simulink library "Pitch_Functions"  (Simulink 6.5)
undefined symbols (not defined in the file or in its folder): A, ABS, B, C, D, P_PitchProfilerAccLim, P_PitchProfilerMaxGain, P_PitchProfilerPostDelay, P_PitchProfilerPreDelay, P_PitchProfilerSpdLim, P_PitchProfilerTc, P_PitchProfilerTcRatio, P_PitchSpinningPos, PITCH_CYCLE_TIME, RND, SQR
libraries: StandardLib x187, WindLib x15, Pitch_Functions x6, simulink x4
(part 3 of 3)

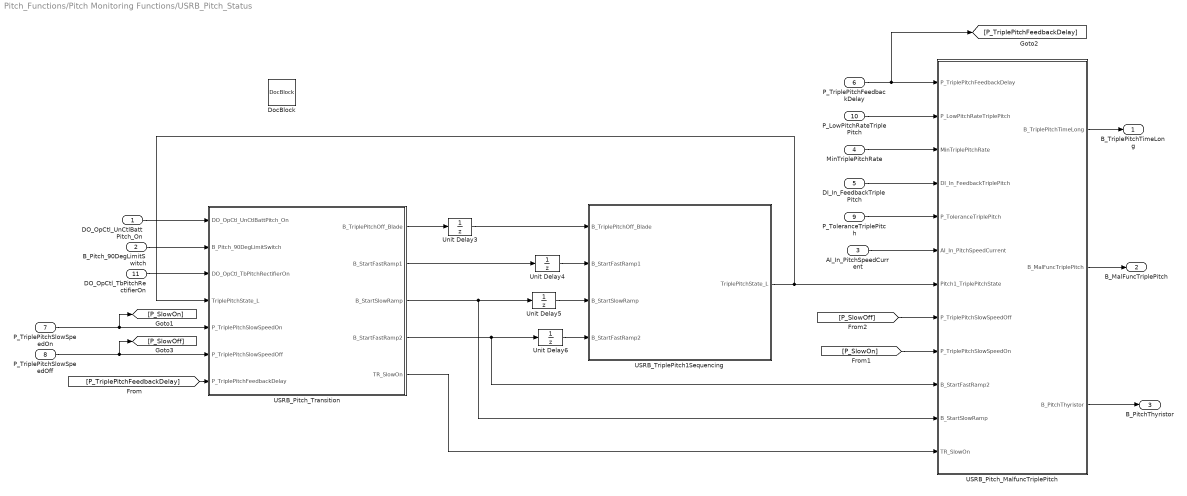
== system Pitch_Functions/Pitch Monitoring Functions/USRB_Pitch_Status ==
  DO_OpCtl_UnCtlBattPitch_On : Inport  DataType=boolean
  B_Pitch_90DegLimitSwitch : Inport  Port=2  DataType=boolean
  AI_In_PitchSpeedCurrent : Inport  Port=3  DataType=single
  MinTriplePitchRate : Inport  Port=4  DataType=single
  DI_In_FeedbackTriplePitch : Inport  Port=5  DataType=boolean
  P_TriplePitchFeedbackDelay : Inport  Port=6  DataType=uint32
  P_TriplePitchSlowSpeedOn : Inport  Port=7  DataType=uint32
  P_TriplePitchSlowSpeedOff : Inport  Port=8  DataType=uint32
  P_ToleranceTriplePitch : Inport  Port=9  DataType=single
  P_LowPitchRateTriplePitch : Inport  Port=10  DataType=single
  DO_OpCtl_TbPitchRectifierOn : Inport  Port=11  DataType=boolean
  DocBlock : simulink/Model-Wide Utilities/DocBlock  SystemSampleTime=-1  DocumentType=Text
  USRB_Pitch_MalfuncTriplePitch : Subsystem  TreatAsAtomicUnit=on
  USRB_Pitch_Transition : Subsystem  TreatAsAtomicUnit=on
  USRB_TriplePitch1Sequencing : Stateflow chart  TreatAsAtomicUnit=on
  Unit Delay{3..6} (4 alike) : UnitDelay  SampleTime=-1
  B_TriplePitchTimeLong : Outport  DataType=boolean
  B_MalFuncTriplePitch : Outport  Port=2  DataType=boolean
  B_PitchThyristor : Outport  Port=3  DataType=boolean
  wires:
  DO_OpCtl_UnCtlBattPitch_On/1 -> USRB_Pitch_Transition/1(DO_OpCtl_UnCtlBattPitch_On)
  B_Pitch_90DegLimitSwitch/1 -> USRB_Pitch_Transition/2(B_Pitch_90DegLimitSwitch)
  DO_OpCtl_TbPitchRectifierOn/1 -> USRB_Pitch_Transition/3(DO_OpCtl_TbPitchRectifierOn)
  P_TriplePitchSlowSpeedOn/1 -> USRB_Pitch_Transition/5(P_TriplePitchSlowSpeedOn), [P_SlowOn]
  P_TriplePitchSlowSpeedOff/1 -> USRB_Pitch_Transition/6(P_TriplePitchSlowSpeedOff), [P_SlowOff]
  MinTriplePitchRate/1 -> USRB_Pitch_MalfuncTriplePitch/3(MinTriplePitchRate)
  AI_In_PitchSpeedCurrent/1 -> USRB_Pitch_MalfuncTriplePitch/6(AI_In_PitchSpeedCurrent)
  P_LowPitchRateTriplePitch/1 -> USRB_Pitch_MalfuncTriplePitch/2(P_LowPitchRateTriplePitch)
  DI_In_FeedbackTriplePitch/1 -> USRB_Pitch_MalfuncTriplePitch/4(DI_In_FeedbackTriplePitch)
  P_ToleranceTriplePitch/1 -> USRB_Pitch_MalfuncTriplePitch/5(P_ToleranceTriplePitch)
  USRB_Pitch_Transition/2(B_StartFastRamp1) -> Unit Delay4/1
  USRB_Pitch_Transition/3(B_StartSlowRamp) -> USRB_Pitch_MalfuncTriplePitch/11(B_StartSlowRamp), Unit Delay5/1
  USRB_TriplePitch1Sequencing/1(TriplePitchState_L) -> USRB_Pitch_Transition/4(TriplePitchState_L), USRB_Pitch_MalfuncTriplePitch/7(Pitch1_TriplePitchState)
  USRB_Pitch_Transition/4(B_StartFastRamp2) -> USRB_Pitch_MalfuncTriplePitch/10(B_StartFastRamp2), Unit Delay6/1
  [P_TriplePitchFeedbackDelay] -> USRB_Pitch_Transition/7(P_TriplePitchFeedbackDelay)
  [P_SlowOn] -> USRB_Pitch_MalfuncTriplePitch/9(P_TriplePitchSlowSpeedOn)
  [P_SlowOff] -> USRB_Pitch_MalfuncTriplePitch/8(P_TriplePitchSlowSpeedOff)
  USRB_Pitch_MalfuncTriplePitch/1(B_TriplePitchTimeLong) -> B_TriplePitchTimeLong/1
  USRB_Pitch_MalfuncTriplePitch/2(B_MalFuncTriplePitch) -> B_MalFuncTriplePitch/1
  USRB_Pitch_MalfuncTriplePitch/3(B_PitchThyristor) -> B_PitchThyristor/1
  P_TriplePitchFeedbackDelay/1 -> USRB_Pitch_MalfuncTriplePitch/1(P_TriplePitchFeedbackDelay), [P_TriplePitchFeedbackDelay]
  USRB_Pitch_Transition/5(TR_SlowOn) -> USRB_Pitch_MalfuncTriplePitch/12(TR_SlowOn)
  Unit Delay4/1 -> USRB_TriplePitch1Sequencing/2(B_StartFastRamp1)
  Unit Delay5/1 -> USRB_TriplePitch1Sequencing/3(B_StartSlowRamp)
  Unit Delay6/1 -> USRB_TriplePitch1Sequencing/4(B_StartFastRamp2)
  USRB_Pitch_Transition/1(B_TriplePitchOff_Blade) -> Unit Delay3/1
  Unit Delay3/1 -> USRB_TriplePitch1Sequencing/1(B_TriplePitchOff_Blade)

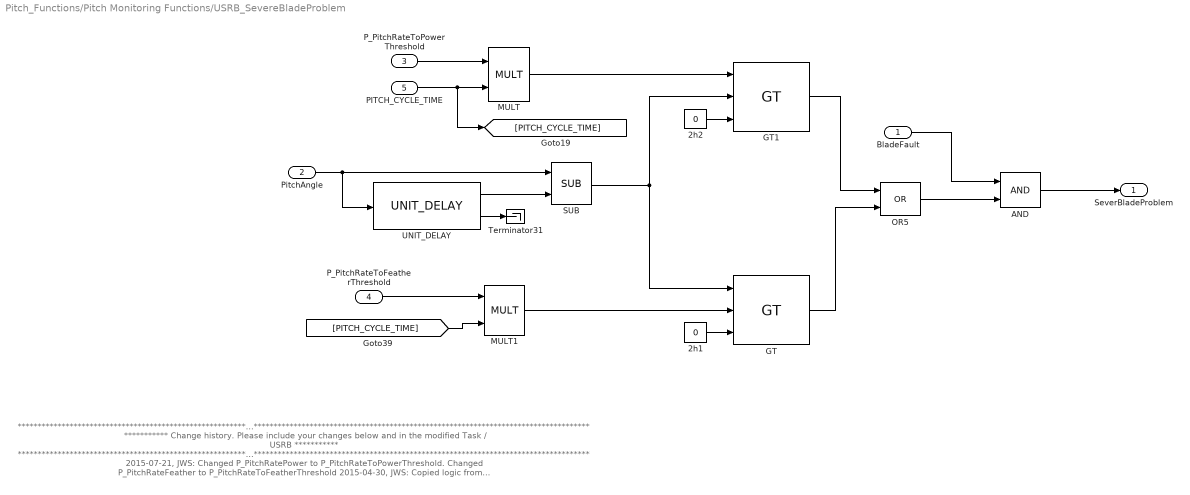
== system Pitch_Functions/Pitch Monitoring Functions/USRB_SevereBladeProblem ==
  note: ***********************************************************************************************************************************************
      | ***********         Change history. Please include your changes below and in the modified Task / USRB         ***********
      | ***********************************************************************************************************************************************
      | 2015-07-21, JWS: Changed P_PitchRatePower to P_PitchRateToPowerThreshold.
      |                             Changed P_PitchRateFeather to P_PitchRateToFeatherThreshold
      | 2015-04-30, JWS: Copied logic from Pitch_TASK_Libs.  Replaced PITCH_CYCLE_TIME constant with input.
      |                               Swapped intputs into SUB block.
  BladeFault : Inport  DataType=boolean
  PitchAngle : Inport  Port=2  DataType=single
  P_PitchRateToPowerThreshold : Inport  Port=3  DataType=single
  P_PitchRateToFeatherThreshold : Inport  Port=4  DataType=single
  PITCH_CYCLE_TIME : Inport  Port=5  DataType=single
  2h1 : Constant  Value=0  OutDataTypeMode=single  OutDataType=sfix(16)  ConRadixGroup=Use specified scaling  OutScaling=2^0  SampleTime=inf  FramePeriod=inf
  2h2 : Constant  Value=0  OutDataTypeMode=single  OutDataType=sfix(16)  ConRadixGroup=Use specified scaling  OutScaling=2^0  SampleTime=inf  FramePeriod=inf
  AND : StandardLib/Logical operations/AND  RepeatCnt=1  SampleTime=-1  ExecutionOrder=0
  GT : StandardLib/Math operations/GT  Equation=>  DataType=SINGLE  SampleTime=-1  ExecutionOrder=0
  GT1 : StandardLib/Math operations/GT  Equation=>  DataType=SINGLE  SampleTime=-1  ExecutionOrder=0
  MULT : StandardLib/Math operations/MULT  DataType=SINGLE  RepeatCnt=1  SampleTime=-1  ExecutionOrder=0
  MULT1 : StandardLib/Math operations/MULT  DataType=SINGLE  RepeatCnt=1  SampleTime=-1  ExecutionOrder=0
  OR5 : StandardLib/Logical operations/OR  RepeatCnt=1  SampleTime=-1  ExecutionOrder=0
  SUB : StandardLib/Math operations/SUB  DataType=SINGLE  SampleTime=-1  ExecutionOrder=0
  Terminator31 : Terminator
  UNIT_DELAY : StandardLib/Memory operations/UNIT_DELAY  DataType=SINGLE  SampleTime=-1  ExecutionOrder=0
  SeverBladeProblem : Outport  DataType=boolean
  wires:
  MULT/1 -> GT1/1
  OR5/1 -> AND/2
  BladeFault/1 -> AND/1
  AND/1 -> SeverBladeProblem/1
  GT1/1 -> OR5/1
  GT/1 -> OR5/2
  SUB/1 -> GT/1, GT1/2
  P_PitchRateToPowerThreshold/1 -> MULT/1
  P_PitchRateToFeatherThreshold/1 -> MULT1/1
  MULT1/1 -> GT/2
  PitchAngle/1 -> SUB/1, UNIT_DELAY/1
  UNIT_DELAY/1 -> SUB/2
  UNIT_DELAY/2 -> Terminator31/1
  PITCH_CYCLE_TIME/1 -> MULT/2, [PITCH_CYCLE_TIME]
  [PITCH_CYCLE_TIME] -> MULT1/2
  2h1/1 -> GT/3
  2h2/1 -> GT1/3

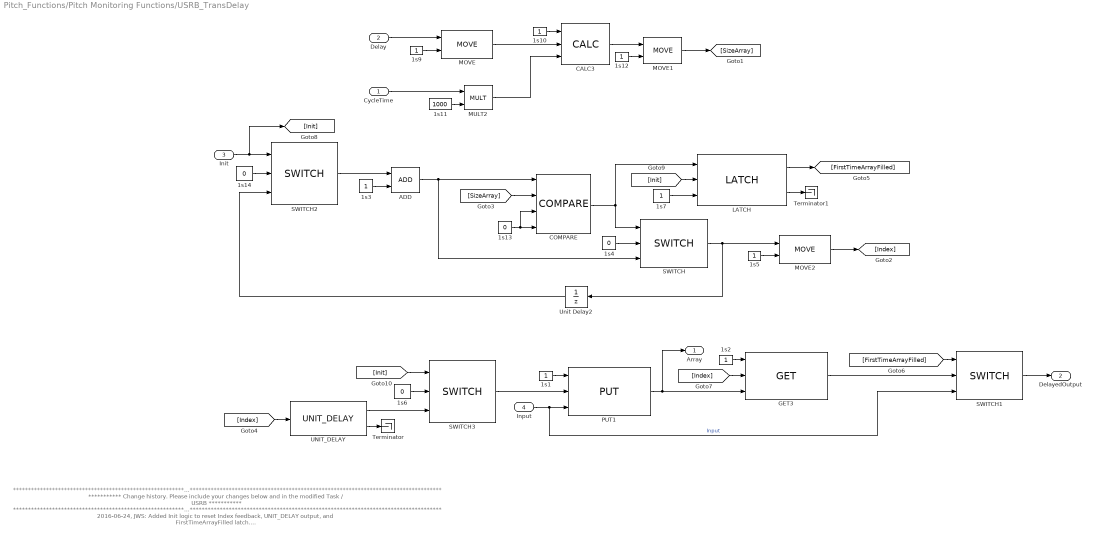
== system Pitch_Functions/Pitch Monitoring Functions/USRB_TransDelay ==
  note: ***********************************************************************************************************************************************
      | ***********         Change history. Please include your changes below and in the modified Task / USRB         ***********
      | ***********************************************************************************************************************************************
      | 2016-06-24, JWS: Added Init logic to reset Index feedback, UNIT_DELAY output, and FirstTimeArrayFilled latch.
      | ***********************************************************************************************************************************************
  CycleTime : Inport  DataType=single
  Delay : Inport  Port=2  DataType=uint32
  Init : Inport  Port=3  DataType=boolean
  Input : Inport  Port=4  DataType=single
  1s{1..2,5,7,9..10,12} (7 alike) : Constant  Value=1  OutDataTypeMode=boolean  OutDataType=sfix(16)  ConRadixGroup=Use specified scaling  OutScaling=2^0  SampleTime=inf  FramePeriod=inf
  1s11 : Constant  Value=1000  OutDataTypeMode=single  OutDataType=sfix(16)  ConRadixGroup=Use specified scaling  OutScaling=2^0  SampleTime=inf  FramePeriod=inf
  1s13 : Constant  Value=0  OutDataTypeMode=int16  OutDataType=sfix(16)  ConRadixGroup=Use specified scaling  OutScaling=2^0  SampleTime=inf  FramePeriod=inf
  1s14 : Constant  Value=0  OutDataTypeMode=int16  OutDataType=sfix(16)  ConRadixGroup=Use specified scaling  OutScaling=2^0  SampleTime=inf  FramePeriod=inf
  1s3 : Constant  Value=1  OutDataTypeMode=int16  OutDataType=sfix(16)  ConRadixGroup=Use specified scaling  OutScaling=2^0  SampleTime=inf  FramePeriod=inf
  1s4 : Constant  Value=0  OutDataTypeMode=int16  OutDataType=sfix(16)  ConRadixGroup=Use specified scaling  OutScaling=2^0  SampleTime=inf  FramePeriod=inf
  1s6 : Constant  Value=0  OutDataTypeMode=uint32  OutDataType=sfix(16)  ConRadixGroup=Use specified scaling  OutScaling=2^0  SampleTime=inf  FramePeriod=inf
  ADD : StandardLib/Math operations/ADD  DataType=INT16  RepeatCnt=1  SampleTime=-1  ExecutionOrder=0
  CALC3 : StandardLib/Math operations/CALC  DataType=SINGLE  RepeatCount=2  Equation=(A/B)  SampleTime=-1  ExecutionOrder=0
  COMPARE : StandardLib/Math operations/COMPARE  Equation=>  DataType=INT16  SampleTime=-1  ExecutionOrder=0
  GET3 : StandardLib/Memory operations/GET  DataType=SINGLE  SampleTime=-1  ExecutionOrder=0
  LATCH : StandardLib/Logical operations/LATCH  SampleTime=-1  ExecutionOrder=0
  MOVE : StandardLib/Memory operations/MOVE  DataType=SINGLE  SampleTime=-1  ExecutionOrder=0
  MOVE1 : StandardLib/Memory operations/MOVE  DataType=INT16  SampleTime=-1  ExecutionOrder=0
  MOVE2 : StandardLib/Memory operations/MOVE  DataType=UINT32  SampleTime=-1  ExecutionOrder=0
  MULT2 : StandardLib/Math operations/MULT  DataType=SINGLE  RepeatCnt=1  SampleTime=-1  ExecutionOrder=0
  PUT1 : StandardLib/Memory operations/PUT  DataType=SINGLE  ArraySize=40  SampleTime=-1  ExecutionOrder=0
  SWITCH : StandardLib/Memory operations/SWITCH  DataType=INT16  SampleTime=-1  ExecutionOrder=0
  SWITCH1 : StandardLib/Memory operations/SWITCH  DataType=SINGLE  SampleTime=-1  ExecutionOrder=0
  SWITCH2 : StandardLib/Memory operations/SWITCH  DataType=INT16  SampleTime=-1  ExecutionOrder=0
  SWITCH3 : StandardLib/Memory operations/SWITCH  DataType=UINT32  SampleTime=-1  ExecutionOrder=0
  Terminator : Terminator
  Terminator1 : Terminator
  UNIT_DELAY : StandardLib/Memory operations/UNIT_DELAY  DataType=UINT32  SampleTime=-1  ExecutionOrder=0
  Unit Delay2 : UnitDelay  Orientation=left  SampleTime=-1
  Array : Outport  PortDimensions=40  DataType=single
  DelayedOutput : Outport  Port=2  DataType=single
  wires:
  1s10/1 -> CALC3/1
  CALC3/1 -> MOVE1/1
  1s12/1 -> MOVE1/2
  MOVE/1 -> CALC3/2
  Delay/1 -> MOVE/1
  1s9/1 -> MOVE/2
  MOVE1/1 -> [SizeArray]
  1s3/1 -> ADD/2
  ADD/1 -> COMPARE/1, SWITCH/3
  COMPARE/1 -> SWITCH/1, LATCH/1
  1s4/1 -> SWITCH/2
  SWITCH/1 -> MOVE2/1, Unit Delay2/1
  [Index] -> UNIT_DELAY/1
  1s1/1 -> PUT1/1
  1s2/1 -> GET3/1
  GET3/1 -> SWITCH1/2
  SWITCH1/1 -> DelayedOutput/1
  [Init] -> LATCH/2
  1s7/1 -> LATCH/3
  LATCH/1 -> [FirstTimeArrayFilled]
  [FirstTimeArrayFilled] -> SWITCH1/1
  1s5/1 -> MOVE2/2
  MOVE2/1 -> [Index]
  [SizeArray] -> COMPARE/2
  1s11/1 -> MULT2/2
  CycleTime/1 -> MULT2/1
  MULT2/1 -> CALC3/3
  [Index] -> GET3/2
  UNIT_DELAY/2 -> Terminator/1
  PUT1/1 -> GET3/3, Array/1
  Input/1 -> PUT1/3, SWITCH1/3  "Input"
  1s13/1 -> COMPARE/3, COMPARE/4
  LATCH/2 -> Terminator1/1
  Init/1 -> SWITCH2/1, [Init]
  1s14/1 -> SWITCH2/2
  SWITCH2/1 -> ADD/1
  Unit Delay2/1 -> SWITCH2/3
  1s6/1 -> SWITCH3/2
  SWITCH3/1 -> PUT1/2
  [Init] -> SWITCH3/1
  UNIT_DELAY/1 -> SWITCH3/3

== system Pitch_Functions/Pitch Models/USRB_PitchProfiler/USRB_Pitch_AccCalc ==
  note: ***********************************************************************************************************************************************
      | ***********         Change history. Please include your changes below and in the modified Task / USRB         ***********
      | ***********************************************************************************************************************************************
      | 2015-09-11, JWS: Replaced constant blocks with inputs.
      | ***********************************************************************************************************************************************
  P_PitchProfilerTc : Inport  DataType=single
  P_PitchProfilerAccLim : Inport  Port=2  DataType=single
  Spd : Inport  Port=3  DataType=single
  Speed_Pre : Inport  Port=4  DataType=single
  CALC3 : StandardLib/Math operations/CALC  DataType=SINGLE  RepeatCount=3  Equation=(A-B)/C  SampleTime=-1  ExecutionOrder=0
  CLAMP1 : StandardLib/Math operations/CLAMP  DataType=SINGLE  SampleTime=-1  ExecutionOrder=0
  Constant25 : Constant  Value=1  OutDataTypeMode=boolean  OutDataType=sfix(16)  ConRadixGroup=Use specified scaling  OutScaling=2^0  SampleTime=inf  FramePeriod=inf
  Constant26 : Constant  Value=1  OutDataTypeMode=boolean  OutDataType=sfix(16)  ConRadixGroup=Use specified scaling  OutScaling=2^0  SampleTime=inf  FramePeriod=inf
  Constant27 : Constant  Value=-1  OutDataTypeMode=single  OutDataType=sfix(16)  ConRadixGroup=Use specified scaling  OutScaling=2^0  SampleTime=inf  FramePeriod=inf
  MULT4 : StandardLib/Math operations/MULT  DataType=SINGLE  RepeatCnt=1  SampleTime=-1  ExecutionOrder=0
  Terminator : Terminator
  Terminator1 : Terminator
  Acc : Outport  DataType=single
  wires:
  CLAMP1/2 -> Terminator1/1
  CLAMP1/1 -> Terminator/1
  Speed_Pre/1 -> CALC3/3
  Spd/1 -> CALC3/2
  CLAMP1/3 -> Acc/1
  CALC3/1 -> CLAMP1/2
  MULT4/1 -> CLAMP1/4
  Constant27/1 -> MULT4/2
  P_PitchProfilerAccLim/1 -> MULT4/1, CLAMP1/3
  Constant26/1 -> CLAMP1/1
  P_PitchProfilerTc/1 -> CALC3/4
  Constant25/1 -> CALC3/1

== system Pitch_Functions/Pitch Models/USRB_PitchProfiler/USRB_Pitch_ErrorCalc ==
  note: ***********************************************************************************************************************************************
      | ***********         Change history. Please include your changes below and in the modified Task / USRB         ***********
      | ***********************************************************************************************************************************************
      | 2015-09-11, JWS: Replaced constant blocks with inputs.
      | ***********************************************************************************************************************************************
  PosRef : Inport  DataType=single
  P_PitchProfilerTc : Inport  Port=2  DataType=single
  P_PitchProfilerTcRatio : Inport  Port=3  DataType=single
  Position_Pre : Inport  Port=4  DataType=single
  Speed_Pre : Inport  Port=5  DataType=single
  CALC : StandardLib/Math operations/CALC  DataType=SINGLE  RepeatCount=5  Equation=A-(B+C*D*E)  SampleTime=-1  ExecutionOrder=0
  Constant13 : Constant  Value=1  OutDataTypeMode=boolean  OutDataType=sfix(16)  ConRadixGroup=Use specified scaling  OutScaling=2^0  SampleTime=inf  FramePeriod=inf
  ErrPos : Outport  DataType=single
  wires:
  Constant13/1 -> CALC/1
  PosRef/1 -> CALC/2
  Position_Pre/1 -> CALC/3
  Speed_Pre/1 -> CALC/4
  CALC/1 -> ErrPos/1
  P_PitchProfilerTc/1 -> CALC/5
  P_PitchProfilerTcRatio/1 -> CALC/6

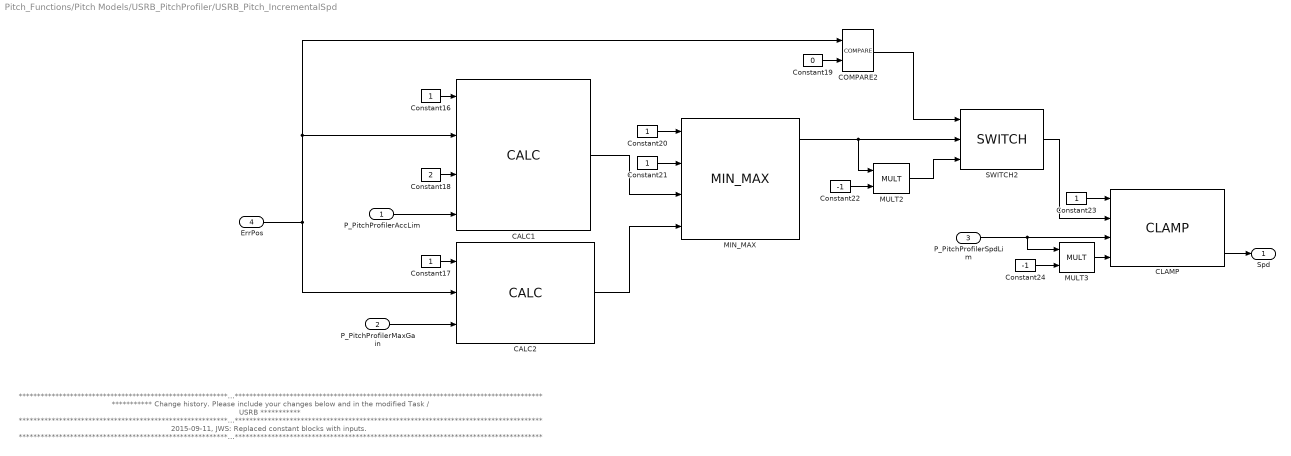
== system Pitch_Functions/Pitch Models/USRB_PitchProfiler/USRB_Pitch_IncrementalSpd ==
  note: ***********************************************************************************************************************************************
      | ***********         Change history. Please include your changes below and in the modified Task / USRB         ***********
      | ***********************************************************************************************************************************************
      | 2015-09-11, JWS: Replaced constant blocks with inputs.
      | ***********************************************************************************************************************************************
  P_PitchProfilerAccLim : Inport  DataType=single
  P_PitchProfilerMaxGain : Inport  Port=2  DataType=single
  P_PitchProfilerSpdLim : Inport  Port=3  DataType=single
  ErrPos : Inport  Port=4  DataType=single
  CALC1 : StandardLib/Math operations/CALC  DataType=SINGLE  RepeatCount=3  Equation=SQR(ABS(A)*B*C)  SampleTime=-1  ExecutionOrder=0
  CALC2 : StandardLib/Math operations/CALC  DataType=SINGLE  RepeatCount=2  Equation=ABS(A)*B  SampleTime=-1  ExecutionOrder=0
  CLAMP : StandardLib/Math operations/CLAMP  DataType=SINGLE  SampleTime=-1  ExecutionOrder=0
  COMPARE2 : StandardLib/Math operations/COMPARE  Equation=>  DataType=SINGLE  SampleTime=-1  ExecutionOrder=0
  Constant{16..17,20,23} (4 alike) : Constant  Value=1  OutDataTypeMode=boolean  OutDataType=sfix(16)  ConRadixGroup=Use specified scaling  OutScaling=2^0  SampleTime=inf  FramePeriod=inf
  Constant18 : Constant  Value=2  OutDataTypeMode=single  OutDataType=sfix(16)  ConRadixGroup=Use specified scaling  OutScaling=2^0  SampleTime=inf  FramePeriod=inf
  Constant19 : Constant  Value=0  OutDataTypeMode=single  OutDataType=sfix(16)  ConRadixGroup=Use specified scaling  OutScaling=2^0  SampleTime=inf  FramePeriod=inf
  Constant21 : Constant  Value=1  OutDataTypeMode=int16  OutDataType=sfix(16)  ConRadixGroup=Use specified scaling  OutScaling=2^0  SampleTime=inf  FramePeriod=inf
  Constant22 : Constant  Value=-1  OutDataTypeMode=single  OutDataType=sfix(16)  ConRadixGroup=Use specified scaling  OutScaling=2^0  SampleTime=inf  FramePeriod=inf
  Constant24 : Constant  Value=-1  OutDataTypeMode=single  OutDataType=sfix(16)  ConRadixGroup=Use specified scaling  OutScaling=2^0  SampleTime=inf  FramePeriod=inf
  MIN_MAX : StandardLib/Math operations/MIN_MAX  RepeatCnt=2  SampleTime=-1  ExecutionOrder=0
  MULT2 : StandardLib/Math operations/MULT  DataType=SINGLE  RepeatCnt=1  SampleTime=-1  ExecutionOrder=0
  MULT3 : StandardLib/Math operations/MULT  DataType=SINGLE  RepeatCnt=1  SampleTime=-1  ExecutionOrder=0
  SWITCH2 : StandardLib/Memory operations/SWITCH  DataType=SINGLE  SampleTime=-1  ExecutionOrder=0
  Spd : Outport  DataType=single
  wires:
  CLAMP/3 -> Spd/1
  SWITCH2/1 -> CLAMP/2
  ErrPos/1 -> COMPARE2/1, CALC1/2, CALC2/2
  MULT3/1 -> CLAMP/4
  Constant24/1 -> MULT3/2
  P_PitchProfilerSpdLim/1 -> CLAMP/3, MULT3/1
  Constant23/1 -> CLAMP/1
  MULT2/1 -> SWITCH2/3
  Constant22/1 -> MULT2/2
  MIN_MAX/1 -> SWITCH2/2, MULT2/1
  CALC2/1 -> MIN_MAX/4
  CALC1/1 -> MIN_MAX/3
  Constant21/1 -> MIN_MAX/2
  Constant20/1 -> MIN_MAX/1
  COMPARE2/1 -> SWITCH2/1
  Constant19/1 -> COMPARE2/2
  P_PitchProfilerAccLim/1 -> CALC1/4
  Constant18/1 -> CALC1/3
  P_PitchProfilerMaxGain/1 -> CALC2/3
  Constant17/1 -> CALC2/1
  Constant16/1 -> CALC1/1

== system Pitch_Functions/Pitch Models/USRB_PitchProfiler/USRB_Pitch_PosCalc ==
  note: ***********************************************************************************************************************************************
      | ***********         Change history. Please include your changes below and in the modified Task / USRB         ***********
      | ***********************************************************************************************************************************************
      | 2015-09-11, JWS: Replaced constant blocks with inputs.
      | ***********************************************************************************************************************************************
  CYCLE_TIME : Inport  DataType=single
  Speed : Inport  Port=2  DataType=single
  Position_Pre : Inport  Port=3  DataType=single
  CALC5 : StandardLib/Math operations/CALC  DataType=SINGLE  RepeatCount=3  Equation=A+B*C  SampleTime=-1  ExecutionOrder=0
  Constant29 : Constant  Value=1  OutDataTypeMode=boolean  OutDataType=sfix(16)  ConRadixGroup=Use specified scaling  OutScaling=2^0  SampleTime=inf  FramePeriod=inf
  Position : Outport  DataType=single
  wires:
  Speed/1 -> CALC5/3
  CALC5/1 -> Position/1  "Position"
  Position_Pre/1 -> CALC5/2
  CYCLE_TIME/1 -> CALC5/4
  Constant29/1 -> CALC5/1

== system Pitch_Functions/Pitch Models/USRB_PitchProfiler/USRB_Pitch_SpeedCalc ==
  note: ***********************************************************************************************************************************************
      | ***********         Change history. Please include your changes below and in the modified Task / USRB         ***********
      | ***********************************************************************************************************************************************
      | 2015-09-11, JWS: Replaced constant blocks with inputs.
      | ***********************************************************************************************************************************************
  CYCLE_TIME : Inport  DataType=single
  Acc : Inport  Port=2  DataType=single
  Speed_Pre : Inport  Port=3  DataType=single
  CALC4 : StandardLib/Math operations/CALC  DataType=SINGLE  RepeatCount=3  Equation=A+B*C  SampleTime=-1  ExecutionOrder=0
  Constant28 : Constant  Value=1  OutDataTypeMode=boolean  OutDataType=sfix(16)  ConRadixGroup=Use specified scaling  OutScaling=2^0  SampleTime=inf  FramePeriod=inf
  Speed : Outport  DataType=single
  wires:
  Acc/1 -> CALC4/3
  Speed_Pre/1 -> CALC4/2
  CALC4/1 -> Speed/1  "Speed"
  CYCLE_TIME/1 -> CALC4/4
  Constant28/1 -> CALC4/1

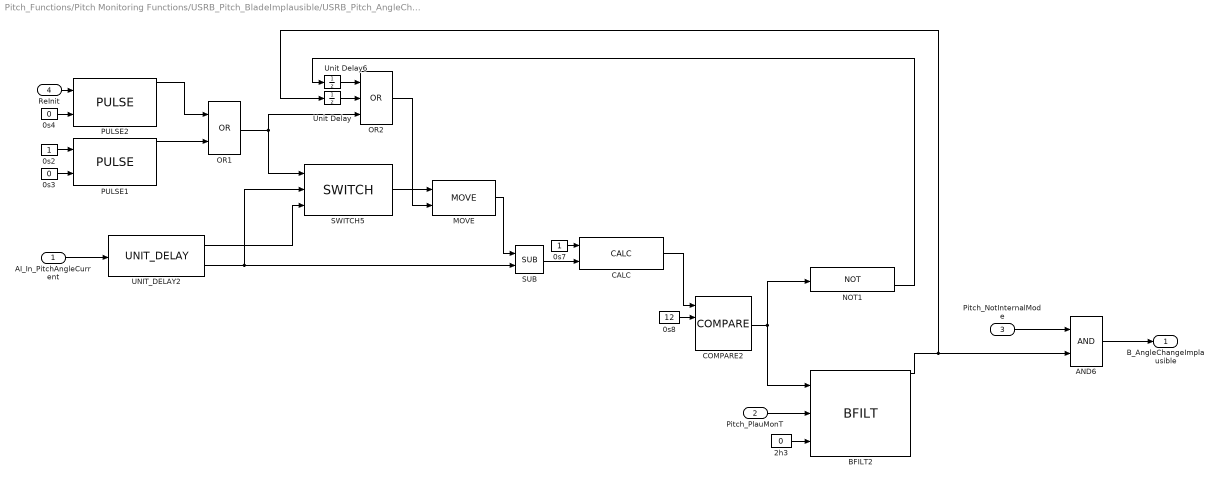
== system Pitch_Functions/Pitch Monitoring Functions/USRB_Pitch_BladeImplausible/USRB_Pitch_AngleChangeCheck ==
  AI_In_PitchAngleCurrent : Inport  DataType=single
  Pitch_PlauMonT : Inport  Port=2  DataType=uint32
  Pitch_NotInternalMode : Inport  Port=3  DataType=boolean
  ReInit : Inport  Port=4  DataType=boolean
  0s2 : Constant  Value=1  OutDataTypeMode=boolean  OutDataType=sfix(16)  ConRadixGroup=Use specified scaling  OutScaling=2^0  SampleTime=inf  FramePeriod=inf
  0s3 : Constant  Value=0  OutDataTypeMode=uint32  OutDataType=sfix(16)  ConRadixGroup=Use specified scaling  OutScaling=2^0  SampleTime=inf  FramePeriod=inf
  0s4 : Constant  Value=0  OutDataTypeMode=uint32  OutDataType=sfix(16)  ConRadixGroup=Use specified scaling  OutScaling=2^0  SampleTime=inf  FramePeriod=inf
  0s7 : Constant  Value=1  OutDataTypeMode=boolean  OutDataType=sfix(16)  ConRadixGroup=Use specified scaling  OutScaling=2^0  SampleTime=inf  FramePeriod=inf
  0s8 : Constant  Value=12  OutDataTypeMode=single  OutDataType=sfix(16)  ConRadixGroup=Use specified scaling  OutScaling=2^0  SampleTime=inf  FramePeriod=inf
  2h3 : Constant  Value=0  OutDataTypeMode=uint32  OutDataType=sfix(16)  ConRadixGroup=Use specified scaling  OutScaling=2^0  SampleTime=inf  FramePeriod=inf
  AND6 : StandardLib/Logical operations/AND  RepeatCnt=1  SampleTime=-1  ExecutionOrder=0
  BFILT2 : StandardLib/Filters/BFILT  SampleTime=-1  ExecutionOrder=0
  CALC : StandardLib/Math operations/CALC  DataType=SINGLE  RepeatCount=1  Equation=ABS(A)  SampleTime=-1  ExecutionOrder=0
  COMPARE2 : StandardLib/Math operations/COMPARE  Equation=>  DataType=SINGLE  SampleTime=-1  ExecutionOrder=0
  MOVE : StandardLib/Memory operations/MOVE  DataType=SINGLE  SampleTime=-1  ExecutionOrder=0
  NOT1 : StandardLib/Logical operations/NOT  SampleTime=-1  ExecutionOrder=0
  OR1 : StandardLib/Logical operations/OR  RepeatCnt=1  SampleTime=-1  ExecutionOrder=0
  OR2 : StandardLib/Logical operations/OR  RepeatCnt=2  SampleTime=-1  ExecutionOrder=0
  PULSE1 : StandardLib/Sequencing/PULSE  SampleTime=-1  ExecutionOrder=0
  PULSE2 : StandardLib/Sequencing/PULSE  SampleTime=-1  ExecutionOrder=0
  SUB : StandardLib/Math operations/SUB  DataType=SINGLE  SampleTime=-1  ExecutionOrder=0
  SWITCH5 : StandardLib/Memory operations/SWITCH  DataType=SINGLE  SampleTime=-1  ExecutionOrder=0
  UNIT_DELAY2 : StandardLib/Memory operations/UNIT_DELAY  DataType=SINGLE  SampleTime=-1  ExecutionOrder=0
  Unit Delay : UnitDelay  SampleTime=-1
  Unit Delay6 : UnitDelay  SampleTime=-1
  B_AngleChangeImplausible : Outport  DataType=boolean
  wires:
  Pitch_NotInternalMode/1 -> AND6/1
  COMPARE2/1 -> NOT1/1, BFILT2/1
  UNIT_DELAY2/1 -> SWITCH5/3
  SWITCH5/1 -> MOVE/1
  UNIT_DELAY2/2 -> SUB/2, SWITCH5/2
  AI_In_PitchAngleCurrent/1 -> UNIT_DELAY2/1
  Pitch_PlauMonT/1 -> BFILT2/2
  NOT1/2 -> Unit Delay6/1
  OR2/1 -> MOVE/2
  BFILT2/1 -> Unit Delay/1, AND6/2
  2h3/1 -> BFILT2/3
  0s8/1 -> COMPARE2/2
  CALC/1 -> COMPARE2/1
  0s7/1 -> CALC/1
  SUB/1 -> CALC/2
  MOVE/1 -> SUB/1
  Unit Delay6/1 -> OR2/1
  Unit Delay/1 -> OR2/2
  AND6/1 -> B_AngleChangeImplausible/1
  0s3/1 -> PULSE1/2
  0s2/1 -> PULSE1/1
  PULSE1/1 -> OR1/2
  OR1/1 -> SWITCH5/1, OR2/3
  0s4/1 -> PULSE2/2
  ReInit/1 -> PULSE2/1
  PULSE2/1 -> OR1/1

== system Pitch_Functions/Pitch Monitoring Functions/USRB_Pitch_BladeImplausible/USRB_Pitch_MinMaxCheck ==
  MinPitchDegree : Inport  DataType=single
  MaxPitchDegree : Inport  Port=2  DataType=single
  Pitch_OORCheckEn : Inport  Port=3  DataType=boolean
  Pitch_PlauMonT : Inport  Port=4  DataType=uint32
  AI_In_PitchAngleCurrent : Inport  Port=5  DataType=single
  2h4 : Constant  Value=0  OutDataTypeMode=uint32  OutDataType=sfix(16)  ConRadixGroup=Use specified scaling  OutScaling=2^0  SampleTime=inf  FramePeriod=inf
  AND11 : StandardLib/Logical operations/AND  RepeatCnt=1  SampleTime=-1  ExecutionOrder=0
  BFILT3 : StandardLib/Filters/BFILT  SampleTime=-1  ExecutionOrder=0
  COMPARE1 : StandardLib/Math operations/COMPARE  Equation=<  DataType=SINGLE  SampleTime=-1  ExecutionOrder=0
  COMPARE9 : StandardLib/Math operations/COMPARE  Equation=<  DataType=SINGLE  SampleTime=-1  ExecutionOrder=0
  OR5 : StandardLib/Logical operations/OR  RepeatCnt=1  SampleTime=-1  ExecutionOrder=0
  B_BladeOusideLimits : Outport  DataType=boolean
  wires:
  OR5/1 -> AND11/2
  AND11/1 -> BFILT3/1
  Pitch_OORCheckEn/1 -> AND11/1
  Pitch_PlauMonT/1 -> BFILT3/2
  2h4/1 -> BFILT3/3
  COMPARE1/1 -> OR5/1
  COMPARE9/1 -> OR5/2
  AI_In_PitchAngleCurrent/1 -> COMPARE9/1, COMPARE1/2
  MaxPitchDegree/1 -> COMPARE1/1
  MinPitchDegree/1 -> COMPARE9/2
  BFILT3/1 -> B_BladeOusideLimits/1

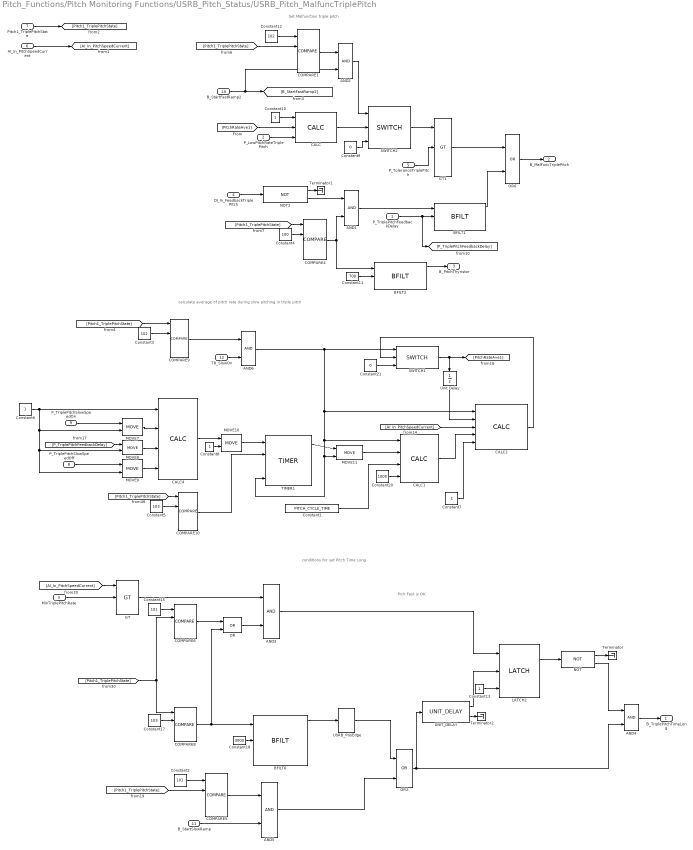
== system Pitch_Functions/Pitch Monitoring Functions/USRB_Pitch_Status/USRB_Pitch_MalfuncTriplePitch ==
  note: Pich Fast is OK
  note: conditions for set Pitch Time Long
  note: Set Malfunction triple pitch
  note: calculate average of pitch rate
      |  during slow pitching in triple pitch
  P_TriplePitchFeedbackDelay : Inport  DataType=uint32
  P_LowPitchRateTriplePitch : Inport  Port=2  DataType=single
  MinTriplePitchRate : Inport  Port=3  DataType=single
  DI_In_FeedbackTriplePitch : Inport  Port=4  DataType=boolean
  P_ToleranceTriplePitch : Inport  Port=5  DataType=single
  AI_In_PitchSpeedCurrent : Inport  Port=6  DataType=single
  Pitch1_TriplePitchState : Inport  Port=7  DataType=int16
  P_TriplePitchSlowSpeedOff : Inport  Port=8  DataType=uint32
  P_TriplePitchSlowSpeedOn : Inport  Port=9  DataType=uint32
  B_StartFastRamp2 : Inport  Port=10  DataType=boolean
  B_StartSlowRamp : Inport  Port=11  DataType=boolean
  TR_SlowOn : Inport  Port=12  DataType=boolean
  AND{1..6} (6 alike) : StandardLib/Logical operations/AND  RepeatCnt=1  SampleTime=-1  ExecutionOrder=0
  BFILT1 : StandardLib/Filters/BFILT  SampleTime=-1  ExecutionOrder=0
  BFILT2 : StandardLib/Filters/BFILT  SampleTime=-1  ExecutionOrder=0
  BFILT6 : StandardLib/Filters/BFILT  SampleTime=-1  ExecutionOrder=0
  CALC : StandardLib/Math operations/CALC  DataType=SINGLE  RepeatCount=2  Equation=ABS(A-B)  SampleTime=-1  ExecutionOrder=0
  CALC1 : StandardLib/Math operations/CALC  DataType=SINGLE  RepeatCount=3  Equation=RND(A/B/C)  SampleTime=-1  ExecutionOrder=0
  CALC2 : StandardLib/Math operations/CALC  DataType=SINGLE  RepeatCount=4  Equation=(A*(C-D)+B)/C  SampleTime=-1  ExecutionOrder=0
  CALC4 : StandardLib/Math operations/CALC  DataType=INT32  RepeatCount=3  Equation=C-A-B  SampleTime=-1  ExecutionOrder=0
  COMPARE{1,5..6,8..10} (6 alike) : StandardLib/Math operations/COMPARE  Equation===  DataType=INT16  SampleTime=-1  ExecutionOrder=0
  COMPARE4 : StandardLib/Math operations/COMPARE  Equation=>  DataType=INT16  SampleTime=-1  ExecutionOrder=0
  Constant1 : Constant  Value=PITCH_CYCLE_TIME  OutDataTypeMode=single  OutDataType=sfix(16)  ConRadixGroup=Use specified scaling  OutScaling=2^0  SampleTime=inf  FramePeriod=inf
  Constant{6,8,10,13} (4 alike) : Constant  Value=1  OutDataTypeMode=boolean  OutDataType=sfix(16)  ConRadixGroup=Use specified scaling  OutScaling=2^0  SampleTime=inf  FramePeriod=inf
  Constant11 : Constant  Value=700  OutDataTypeMode=uint32  OutDataType=sfix(16)  ConRadixGroup=Use specified scaling  OutScaling=2^0  SampleTime=inf  FramePeriod=inf
  Constant12 : Constant  Value=102  OutDataTypeMode=int16  OutDataType=sfix(16)  ConRadixGroup=Use specified scaling  OutScaling=2^0  SampleTime=inf  FramePeriod=inf
  Constant15 : Constant  Value=101  OutDataTypeMode=int16  OutDataType=sfix(16)  ConRadixGroup=Use specified scaling  OutScaling=2^0  SampleTime=inf  FramePeriod=inf
  Constant17 : Constant  Value=103  OutDataTypeMode=int16  OutDataType=sfix(16)  ConRadixGroup=Use specified scaling  OutScaling=2^0  SampleTime=inf  FramePeriod=inf
  Constant18 : Constant  Value=3000  OutDataTypeMode=uint32  OutDataType=sfix(16)  ConRadixGroup=Use specified scaling  OutScaling=2^0  SampleTime=inf  FramePeriod=inf
  Constant2 : Constant  Value=101  OutDataTypeMode=int16  OutDataType=sfix(16)  ConRadixGroup=Use specified scaling  OutScaling=2^0  SampleTime=inf  FramePeriod=inf
  Constant20 : Constant  Value=1000  OutDataTypeMode=single  OutDataType=sfix(16)  ConRadixGroup=Use specified scaling  OutScaling=2^0  SampleTime=inf  FramePeriod=inf
  Constant21 : Constant  Value=0  OutDataTypeMode=single  OutDataType=sfix(16)  ConRadixGroup=Use specified scaling  OutScaling=2^0  SampleTime=inf  FramePeriod=inf
  Constant3 : Constant  Value=102  OutDataTypeMode=int16  OutDataType=sfix(16)  ConRadixGroup=Use specified scaling  OutScaling=2^0  SampleTime=inf  FramePeriod=inf
  Constant4 : Constant  Value=100  OutDataTypeMode=int16  OutDataType=sfix(16)  ConRadixGroup=Use specified scaling  OutScaling=2^0  SampleTime=inf  FramePeriod=inf
  Constant5 : Constant  Value=103  OutDataTypeMode=int16  OutDataType=sfix(16)  ConRadixGroup=Use specified scaling  OutScaling=2^0  SampleTime=inf  FramePeriod=inf
  Constant7 : Constant  Value=1  OutDataTypeMode=single  OutDataType=sfix(16)  ConRadixGroup=Use specified scaling  OutScaling=2^0  SampleTime=inf  FramePeriod=inf
  Constant9 : Constant  Value=0  OutDataTypeMode=single  OutDataType=sfix(16)  ConRadixGroup=Use specified scaling  OutScaling=2^0  SampleTime=inf  FramePeriod=inf
  GT : StandardLib/Math operations/GT  Equation=>  DataType=SINGLE  SampleTime=-1  ExecutionOrder=0
  GT1 : StandardLib/Math operations/GT  Equation=>  DataType=SINGLE  SampleTime=-1  ExecutionOrder=0
  LATCH2 : StandardLib/Logical operations/LATCH  SampleTime=-1  ExecutionOrder=0
  MOVE10 : StandardLib/Memory operations/MOVE  DataType=UINT32  SampleTime=-1  ExecutionOrder=0
  MOVE11 : StandardLib/Memory operations/MOVE  DataType=SINGLE  SampleTime=-1  ExecutionOrder=0
  MOVE7 : StandardLib/Memory operations/MOVE  DataType=INT32  SampleTime=-1  ExecutionOrder=0
  MOVE8 : StandardLib/Memory operations/MOVE  DataType=INT32  SampleTime=-1  ExecutionOrder=0
  MOVE9 : StandardLib/Memory operations/MOVE  DataType=INT32  SampleTime=-1  ExecutionOrder=0
  NOT : StandardLib/Logical operations/NOT  SampleTime=-1  ExecutionOrder=0
  NOT2 : StandardLib/Logical operations/NOT  SampleTime=-1  ExecutionOrder=0
  OR : StandardLib/Logical operations/OR  RepeatCnt=1  SampleTime=-1  ExecutionOrder=0
  OR2 : StandardLib/Logical operations/OR  RepeatCnt=1  SampleTime=-1  ExecutionOrder=0
  OR6 : StandardLib/Logical operations/OR  RepeatCnt=1  SampleTime=-1  ExecutionOrder=0
  SWITCH1 : StandardLib/Memory operations/SWITCH  DataType=SINGLE  SampleTime=-1  ExecutionOrder=0
  SWITCH2 : StandardLib/Memory operations/SWITCH  DataType=SINGLE  SampleTime=-1  ExecutionOrder=0
  TIMER1 : StandardLib/Timers and Counters/TIMER  SampleTime=-1  ExecutionOrder=0
  Terminator : Terminator
  Terminator1 : Terminator
  Terminator2 : Terminator
  UNIT_DELAY : StandardLib/Memory operations/UNIT_DELAY  DataType=BOOLEAN  SampleTime=-1  ExecutionOrder=0
  USRB_PosEdge : WindLib/USRB_PosEdge  SystemSampleTime=-1
  Unit Delay : UnitDelay  Orientation=down  SampleTime=-1
  B_TriplePitchTimeLong : Outport  DataType=boolean
  B_MalFuncTriplePitch : Outport  Port=2  DataType=boolean
  B_PitchThyristor : Outport  Port=3  DataType=boolean
  wires:
  UNIT_DELAY/2 -> Terminator2/1
  UNIT_DELAY/1 -> LATCH2/2
  Constant13/1 -> LATCH2/3
  LATCH2/1 -> NOT/1
  AND3/1 -> LATCH2/1
  OR6/1 -> B_MalFuncTriplePitch/1
  BFILT1/1 -> OR6/2
  P_TriplePitchFeedbackDelay/1 -> BFILT1/2, [P_TriplePitchFeedbackDelay]
  AND1/1 -> BFILT1/1
  NOT2/2 -> AND1/1
  DI_In_FeedbackTriplePitch/1 -> NOT2/1
  AI_In_PitchSpeedCurrent/1 -> [AI_In_PitchSpeedCurrent]
  COMPARE4/1 -> AND1/2, BFILT2/1
  Constant4/1 -> COMPARE4/2
  [Pitch1_TriplePitchState] -> COMPARE4/1
  AND4/1 -> B_TriplePitchTimeLong/1
  OR/1 -> AND3/2
  COMPARE6/1 -> OR/1
  Constant15/1 -> COMPARE6/1
  NOT/2 -> AND4/1
  GT/1 -> AND3/1
  MinTriplePitchRate/1 -> GT/2
  [AI_In_PitchSpeedCurrent] -> GT/1
  Constant17/1 -> COMPARE8/2
  [Pitch1_TriplePitchState] -> COMPARE6/2, COMPARE8/1
  COMPARE8/1 -> OR/2, BFILT6/1
  OR2/1 -> UNIT_DELAY/1, AND4/2
  P_LowPitchRateTriplePitch/1 -> CALC/3
  P_ToleranceTriplePitch/1 -> GT1/2
  [PitchRateAve1] -> CALC/2
  Constant5/1 -> COMPARE10/2
  [Pitch1_TriplePitchState] -> COMPARE10/1
  COMPARE10/1 -> TIMER1/2
  TIMER1/2 -> MOVE11/1
  MOVE11/1 -> CALC1/2
  CALC4/1 -> MOVE10/1
  MOVE10/1 -> TIMER1/1
  Constant8/1 -> MOVE10/2
  MOVE9/1 -> CALC4/4
  [P_TriplePitchFeedbackDelay] -> MOVE8/1
  MOVE8/1 -> CALC4/3
  MOVE7/1 -> CALC4/2
  Constant6/1 -> CALC4/1, MOVE7/2, MOVE9/2, MOVE8/2
  [AI_In_PitchSpeedCurrent] -> CALC2/3
  CALC1/1 -> CALC2/4
  Constant1/1 -> CALC1/3
  Constant20/1 -> CALC1/4
  SWITCH1/1 -> Unit Delay/1, [PitchRateAve1]
  CALC2/1 -> SWITCH1/2
  Constant21/1 -> SWITCH1/3
  Unit Delay/1 -> CALC2/2
  Constant18/1 -> BFILT6/2
  Pitch1_TriplePitchState/1 -> [Pitch1_TriplePitchState]
  [Pitch1_TriplePitchState] -> COMPARE9/1
  Constant3/1 -> COMPARE9/2
  AND6/1 -> SWITCH1/1, TIMER1/4, MOVE11/2, CALC1/1, CALC2/1
  Constant7/1 -> CALC2/5
  Constant11/1 -> BFILT2/2
  BFILT2/1 -> B_PitchThyristor/1
  NOT/1 -> Terminator/1
  NOT2/1 -> Terminator1/1
  COMPARE9/1 -> AND6/1
  TR_SlowOn/1 -> AND6/2
  Constant2/1 -> COMPARE5/1
  [Pitch1_TriplePitchState] -> COMPARE5/2
  COMPARE5/1 -> AND5/1
  AND5/1 -> OR2/2
  B_StartSlowRamp/1 -> AND5/2
  B_StartFastRamp2/1 -> [B_StartFastRamp2], AND2/2
  P_TriplePitchSlowSpeedOn/1 -> MOVE7/1
  P_TriplePitchSlowSpeedOff/1 -> MOVE9/1
  CALC/1 -> SWITCH2/2
  SWITCH2/1 -> GT1/1
  Constant9/1 -> SWITCH2/3
  Constant10/1 -> CALC/1
  GT1/1 -> OR6/1
  Constant12/1 -> COMPARE1/1
  [Pitch1_TriplePitchState] -> COMPARE1/2
  COMPARE1/1 -> AND2/1
  AND2/1 -> SWITCH2/1
  BFILT6/1 -> USRB_PosEdge/1
  USRB_PosEdge/1 -> OR2/1

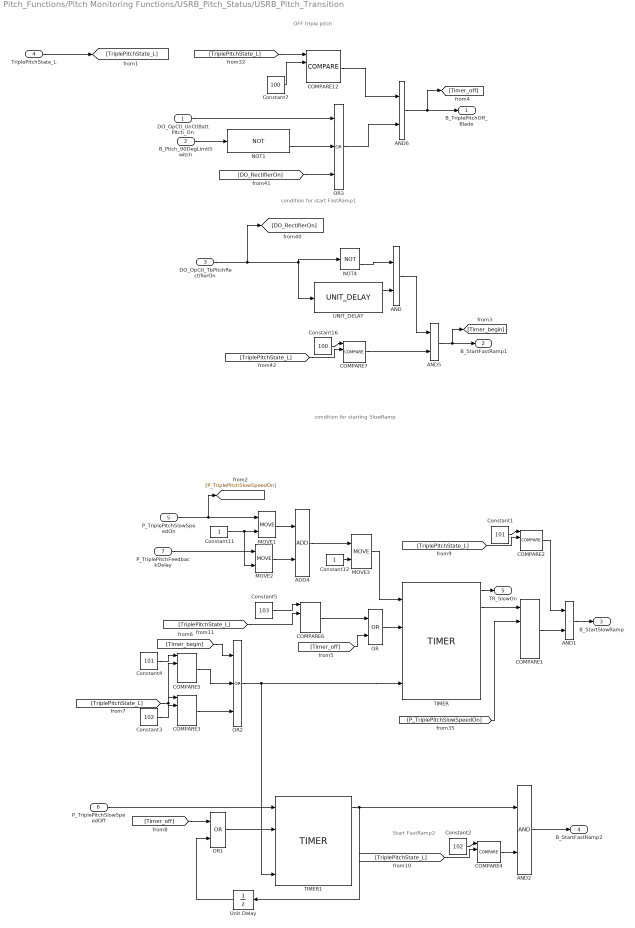
== system Pitch_Functions/Pitch Monitoring Functions/USRB_Pitch_Status/USRB_Pitch_Transition ==
  note: condition for start FastRamp1
  note: Start FastRamp2
  note: condition for starting SlowRamp
  note: OFF triple pitch
  DO_OpCtl_UnCtlBattPitch_On : Inport  DataType=boolean
  B_Pitch_90DegLimitSwitch : Inport  Port=2  DataType=boolean
  DO_OpCtl_TbPitchRectifierOn : Inport  Port=3  DataType=boolean
  TriplePitchState_L : Inport  Port=4  DataType=int16
  P_TriplePitchSlowSpeedOn : Inport  Port=5  DataType=uint32
  P_TriplePitchSlowSpeedOff : Inport  Port=6  DataType=uint32
  P_TriplePitchFeedbackDelay : Inport  Port=7  DataType=uint32
  ADD4 : StandardLib/Math operations/ADD  DataType=INT32  RepeatCnt=1  SampleTime=-1  ExecutionOrder=0
  AND{,1..2,5..6} (5 alike) : StandardLib/Logical operations/AND  RepeatCnt=1  SampleTime=-1  ExecutionOrder=0
  COMPARE1 : StandardLib/Math operations/COMPARE  Equation=>  DataType=UINT32  SampleTime=-1  ExecutionOrder=0
  COMPARE12 : StandardLib/Math operations/COMPARE  Equation=>  DataType=INT16  SampleTime=-1  ExecutionOrder=0
  COMPARE{2..7} (6 alike) : StandardLib/Math operations/COMPARE  Equation===  DataType=INT16  SampleTime=-1  ExecutionOrder=0
  Constant1 : Constant  Value=101  OutDataTypeMode=int16  OutDataType=sfix(16)  ConRadixGroup=Use specified scaling  OutScaling=2^0  SampleTime=inf  FramePeriod=inf
  Constant11 : Constant  Value=1  OutDataTypeMode=boolean  OutDataType=sfix(16)  ConRadixGroup=Use specified scaling  OutScaling=2^0  SampleTime=inf  FramePeriod=inf
  Constant12 : Constant  Value=1  OutDataTypeMode=boolean  OutDataType=sfix(16)  ConRadixGroup=Use specified scaling  OutScaling=2^0  SampleTime=inf  FramePeriod=inf
  Constant16 : Constant  Value=100  OutDataTypeMode=int16  OutDataType=sfix(16)  ConRadixGroup=Use specified scaling  OutScaling=2^0  SampleTime=inf  FramePeriod=inf
  Constant2 : Constant  Value=102  OutDataTypeMode=int16  OutDataType=sfix(16)  ConRadixGroup=Use specified scaling  OutScaling=2^0  SampleTime=inf  FramePeriod=inf
  Constant3 : Constant  Value=102  OutDataTypeMode=int16  OutDataType=sfix(16)  ConRadixGroup=Use specified scaling  OutScaling=2^0  SampleTime=inf  FramePeriod=inf
  Constant4 : Constant  Value=101  OutDataTypeMode=int16  OutDataType=sfix(16)  ConRadixGroup=Use specified scaling  OutScaling=2^0  SampleTime=inf  FramePeriod=inf
  Constant5 : Constant  Value=103  OutDataTypeMode=int16  OutDataType=sfix(16)  ConRadixGroup=Use specified scaling  OutScaling=2^0  SampleTime=inf  FramePeriod=inf
  Constant7 : Constant  Value=100  OutDataTypeMode=int16  OutDataType=sfix(16)  ConRadixGroup=Use specified scaling  OutScaling=2^0  SampleTime=inf  FramePeriod=inf
  MOVE1 : StandardLib/Memory operations/MOVE  DataType=INT32  SampleTime=-1  ExecutionOrder=0
  MOVE2 : StandardLib/Memory operations/MOVE  DataType=INT32  SampleTime=-1  ExecutionOrder=0
  MOVE3 : StandardLib/Memory operations/MOVE  DataType=UINT32  SampleTime=-1  ExecutionOrder=0
  NOT1 : StandardLib/Logical operations/NOT  SampleTime=-1  ExecutionOrder=0
  NOT4 : StandardLib/Logical operations/NOT  SampleTime=-1  ExecutionOrder=0
  OR : StandardLib/Logical operations/OR  RepeatCnt=1  SampleTime=-1  ExecutionOrder=0
  OR1 : StandardLib/Logical operations/OR  RepeatCnt=1  SampleTime=-1  ExecutionOrder=0
  OR2 : StandardLib/Logical operations/OR  RepeatCnt=2  SampleTime=-1  ExecutionOrder=0
  OR3 : StandardLib/Logical operations/OR  RepeatCnt=2  SampleTime=-1  ExecutionOrder=0
  TIMER : StandardLib/Timers and Counters/TIMER  SampleTime=-1  ExecutionOrder=0
  TIMER1 : StandardLib/Timers and Counters/TIMER  SampleTime=-1  ExecutionOrder=0
  UNIT_DELAY : StandardLib/Memory operations/UNIT_DELAY  DataType=BOOLEAN  SampleTime=-1  ExecutionOrder=0
  Unit Delay : UnitDelay  Orientation=left  SampleTime=-1
  B_TriplePitchOff_Blade : Outport  DataType=boolean
  B_StartFastRamp1 : Outport  Port=2  DataType=boolean
  B_StartSlowRamp : Outport  Port=3  DataType=boolean
  B_StartFastRamp2 : Outport  Port=4  DataType=boolean
  TR_SlowOn : Outport  Port=5  DataType=boolean
  wires:
  COMPARE12/1 -> AND6/1
  [TriplePitchState_L] -> COMPARE12/1
  Constant7/1 -> COMPARE12/2
  [DO_RectifierOn] -> OR3/3
  B_Pitch_90DegLimitSwitch/1 -> NOT1/1
  NOT1/2 -> OR3/2
  DO_OpCtl_UnCtlBattPitch_On/1 -> OR3/1
  OR3/1 -> AND6/2
  COMPARE7/1 -> AND5/2
  Constant16/1 -> COMPARE7/1
  AND/1 -> AND5/1
  UNIT_DELAY/1 -> AND/2
  DO_OpCtl_TbPitchRectifierOn/1 -> UNIT_DELAY/1, NOT4/1, [DO_RectifierOn]
  NOT4/2 -> AND/1
  [TriplePitchState_L] -> COMPARE7/2
  Constant12/1 -> MOVE3/2
  ADD4/1 -> MOVE3/1
  MOVE2/1 -> ADD4/2
  MOVE1/1 -> ADD4/1
  Constant11/1 -> MOVE2/2, MOVE1/2
  P_TriplePitchFeedbackDelay/1 -> MOVE2/1
  MOVE3/1 -> TIMER/1
  P_TriplePitchSlowSpeedOn/1 -> MOVE1/1, [P_TriplePitchSlowSpeedOn]
  TIMER/2 -> COMPARE1/1
  [P_TriplePitchSlowSpeedOn] -> COMPARE1/2
  AND6/1 -> B_TriplePitchOff_Blade/1, [Timer_off]
  AND5/1 -> [Timer_begin], B_StartFastRamp1/1
  TriplePitchState_L/1 -> [TriplePitchState_L]
  [TriplePitchState_L] -> COMPARE5/2, COMPARE3/1
  Constant3/1 -> COMPARE3/2
  Constant4/1 -> COMPARE5/1
  [Timer_begin] -> OR2/1
  COMPARE5/1 -> OR2/2
  COMPARE3/1 -> OR2/3
  OR2/1 -> TIMER/4, TIMER1/4
  OR/1 -> TIMER/2
  TIMER1/1 -> Unit Delay/1, AND2/1
  P_TriplePitchSlowSpeedOff/1 -> TIMER1/1
  [Timer_off] -> OR1/1
  OR1/1 -> TIMER1/2
  Unit Delay/1 -> OR1/2
  TIMER/1 -> TR_SlowOn/1
  Constant1/1 -> COMPARE2/1
  [TriplePitchState_L] -> COMPARE2/2
  COMPARE2/1 -> AND1/1
  COMPARE1/1 -> AND1/2
  AND1/1 -> B_StartSlowRamp/1
  Constant2/1 -> COMPARE4/1
  [TriplePitchState_L] -> COMPARE4/2
  AND2/1 -> B_StartFastRamp2/1
  COMPARE4/1 -> AND2/2
  COMPARE6/1 -> OR/1
  [Timer_off] -> OR/2
  Constant5/1 -> COMPARE6/1
  [TriplePitchState_L] -> COMPARE6/2

== stateflow chart Pitch Monitoring Functions/USRB_Pitch_Status/USRB_TriplePitch1Sequencing ==
  state OFF_Pitch
    entry:
    TriplePitchState_L=100;
    during:
    TriplePitchState_L=100;
    exit:
    TriplePitchState_L=100;
  state FastRamp1_Pitch
    entry:
    TriplePitchState_L=101;
    during:
    TriplePitchState_L=101;
    exit:
    TriplePitchState_L=101;
  state FastRamp2_Pitch
    entry:
    TriplePitchState_L=103;
    during:
    TriplePitchState_L=103;
    exit:
    TriplePitchState_L=103;
  state SlowRamp_Pitch
    entry:
    TriplePitchState_L=102;
    during:
    TriplePitchState_L=102;
    exit:
    TriplePitchState_L=102;
  OFF_Pitch -> FastRamp1_Pitch : [B_StartFastRamp1==1]
  FastRamp1_Pitch -> SlowRamp_Pitch [order 2] : [B_StartSlowRamp==1]
  SlowRamp_Pitch -> FastRamp2_Pitch [order 2] : [B_StartFastRamp2==1]
  FastRamp1_Pitch -> OFF_Pitch [order 1] : [B_TriplePitchOff_Blade==1]
  SlowRamp_Pitch -> OFF_Pitch [order 1] : [B_TriplePitchOff_Blade==1]
  FastRamp2_Pitch -> OFF_Pitch : [B_TriplePitchOff_Blade==1]
  (default) -> OFF_Pitch
  data: B_TriplePitchOff_Blade input boolean; B_StartFastRamp1 input boolean; B_StartSlowRamp input boolean; B_StartFastRamp2 input boolean; TriplePitchState_L output int16
